simulink model "WaterTankSysIden2024"  (R2023b)
settings: Solver=FixedStepAuto  StartTime=0.0  StopTime=2000  FixedStep=0.75  RelTol=1e-3  EnableMultiTasking=on
StopFcn:
  | FileName=' SysIdenData00.mat';
  | [fPath, fName, fExt] = fileparts(FileName);
  | if isempty(fExt)  % No '.mat' in FileName
  |     fExt     = '.mat';
  |     FileName = fullfile(fPath, [fName, fExt]);
  | end
  | if exist(FileName, 'file')
  |     % Get number of files:
  |     fDir     = dir(fullfile(fPath, [fName, '*', fExt]));
  |     fStr     = lower(sprintf('%s*', fDir.name));
  |     %fNum     = sscanf(fStr, [fName, '%d', fExt, '*']);
  |     digit =  str2double(extract(fStr, digitsPattern));
  |     %newNum = digit + 1;
  |     if isempty(digit)
  |         newNum = 1;
  |     else
  |         newNum = digit + 1;
  |     end
  |     FileName = fullfile(fPath, [fName, sprintf('%d', newNum(end)), fExt]);
  | end
  | save(FileName, 'LogData');
  | clear digit fDir fExt FileName fName fPath fStr newNum fNum
undefined symbols (not defined in the file or in its folder): National_Instruments, PCIe
libraries: sldrtlib x4, simulink x1
settings Model: SimulationMode=external  ExtModeTrigDuration=7200  ExtModeArchiveMode=auto  ExtModeArchiveFileName=SysIdenData  ExtModeArchiveDirName=C:\Users\My Project\Documents\MATLAB  ExtModeAutoIncOneShot=on  ExtModeWriteAllDataToWs=on  Creator=My Project  LastModifiedBy=My Project
settings SolverCC: AlgebraicLoopSolver=TrustRegion
settings DataIOCC: LimitDataPoints=on  ReturnWorkspaceOutputs=off
settings OptimizationCC: ReuseModelBlockBuffer=off  LifeSpan=inf
settings DebuggingCC: UnconnectedInputMsg=warning  UnconnectedOutputMsg=warning  UnconnectedLineMsg=warning  AllowSymbolicDim=off  SFUnexpectedBacktrackingDiag=warning  SFNoUnconditionalDefaultTransitionDiag=warning  SFExecutionAtInitializationDiag=none  ArithmeticOperatorsInVariantConditions=warning
settings HardwareCC: ProdBitPerLong=64  ProdHWDeviceType=Intel->x86-64 (Linux 64)  TargetBitPerLong=64  TargetBitPerPointer=64  TargetIntDivRoundTo=Zero  TargetEndianess=LittleEndian  TargetWordSize=64  TargetHWDeviceType=Intel->x86-64
settings ModelReferenceCC: EnableRefExpFcnMdlSchedulingChecks=on  PropagateSignalLabelsOutOfModel=off
settings SFSimCC: SimUseLocalCustomCode=off  CustomCodeUndefinedFunction=UseInterfaceOnly
settings RTWCC: Description=Simulink Desktop Real-Time  SystemTargetFile=sldrt.tlc  TemplateMakefile=sldrt.tmf  RTWUseLocalCustomCode=off  RTWCompilerOptimization=on
settings CodeAppCC: MaxIdLength=95  StateflowObjectComments=on
settings SimulinkDesktopRealTimeCC: TargetLibSuffix=_sldrt.a  TargetPreCompLibLocation=C:\Program Files\MATLAB\R2023b\toolbox\sldrt\lib\win64  TargetLangStandard=C89/C90 (ANSI)  SupportVariableSizeSignals=off
settings ConfigComp: CovMetricSettings=dw  CovSaveCumulativeToWorkspaceVar=on  CovSaveSingleToWorkspaceVar=on  CovExternalEMLEnable=off

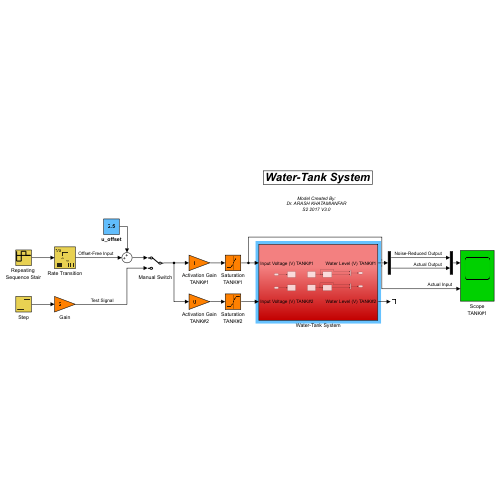
[thumbnail: Simulink's stored preview of the top-level diagram]
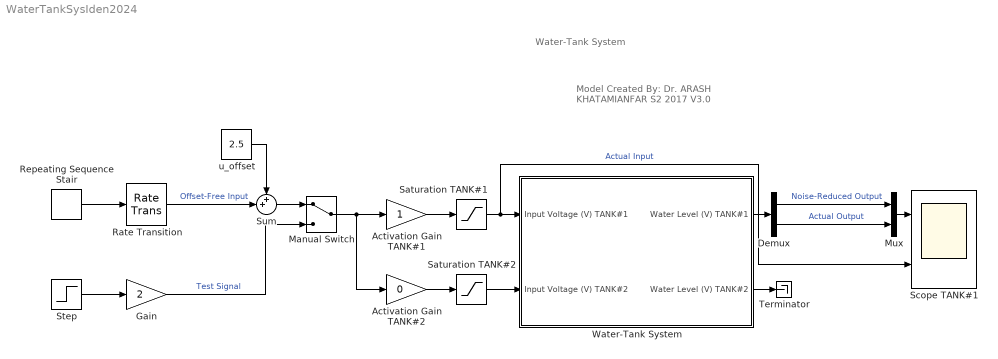
== system WaterTankSysIden2024 ==
  note: Model Created By:
      | Dr. ARASH KHATAMIANFAR
      | S2 2017 V3.0
  note: Water-Tank System
  Activation Gain TANK#1 : Gain
  Activation Gain TANK#2 : Gain  Gain=0
  Demux : Demux  Outputs=2
  Gain : Gain  Gain=2
  Manual Switch : ManualSwitch
  Mux : Mux  Inputs=2
  Rate Transition : RateTransition  OutPortSampleTime=0.75
  Repeating Sequence Stair : simulink/Sources/Repeating Sequence Stair  OutValues=[-0.3 0.2 0].'  tsamp=230*0.75  OutMin=[]  OutMax=[]  OutDataTypeStr=double  OutputDataTypeScalingMode=double  OutDataType=fixdt(0,8)  ConRadixGroup=Best Precision: Vector-wise  OutScaling=2^-12
  Saturation TANK#1 : Saturate  UpperLimit=3  LowerLimit=0
  Saturation TANK#2 : Saturate  UpperLimit=5  LowerLimit=0
  Scope TANK#1 : Scope  NumInputPorts=2
  Step : Step  Time=0  SampleTime=0
  Sum : Sum  Inputs=++|
  Terminator : Terminator
  Water-Tank System : Subsystem
  u_offset : Constant  Value=2.5
  wires:
  Step/1 -> Gain/1
  Repeating Sequence Stair/1 -> Rate Transition/1
  u_offset/1 -> Sum/1
  Sum/1 -> Manual Switch/1
  Saturation TANK#1/1 -> Water-Tank System/1(Input Voltage (V) TANK#1), Scope TANK#1/2  "Actual Input"
  Activation Gain TANK#1/1 -> Saturation TANK#1/1
  Activation Gain TANK#2/1 -> Saturation TANK#2/1
  Saturation TANK#2/1 -> Water-Tank System/2(Input Voltage (V) TANK#2)
  Rate Transition/1 -> Sum/2  "Offset-Free Input"
  Gain/1 -> Manual Switch/2  "Test Signal"
  Manual Switch/1 -> Activation Gain TANK#2/1, Activation Gain TANK#1/1
  Water-Tank System/2(Water Level (V) TANK#2) -> Terminator/1
  Water-Tank System/1(Water Level (V) TANK#1) -> Demux/1
  Demux/2 -> Mux/2  "Actual Output"
  Demux/1 -> Mux/1  "Noise-Reduced Output"
  Mux/1 -> Scope TANK#1/1

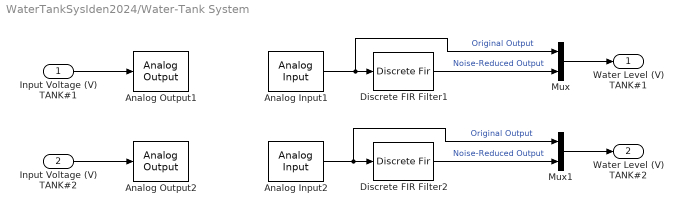
== system WaterTankSysIden2024/Water-Tank System ==
  Input Voltage (V) TANK#1 : Inport
  Input Voltage (V) TANK#2 : Inport  Port=2
  Analog Input1 : sldrtlib/Analog Input  SampleTime=0.75  MaxMissedTicks=10  ShowMissedTicks=off  YieldWhenWaiting=off  DrvName=National_Instruments/PCIe-6351  DrvAddress=4294967295  DrvOptions=[0 0 0 0 0 0 0]  Channels=1  RangeMode=1  VoltRange=1  DataType=1
      settings: AttributesFormatString=National Instruments\nPCIe-6351 [auto]
  Analog Input2 : sldrtlib/Analog Input  SampleTime=0.75  MaxMissedTicks=10  ShowMissedTicks=off  YieldWhenWaiting=off  DrvName=National_Instruments/PCIe-6351  DrvAddress=4294967295  DrvOptions=[0 0 0 0 0 0 0]  Channels=2  RangeMode=1  VoltRange=1  DataType=1
      settings: AttributesFormatString=National Instruments\nPCIe-6351 [auto]
  Analog Output1 : sldrtlib/Analog Output  SampleTime=0.75  MaxMissedTicks=10  ShowMissedTicks=off  YieldWhenWaiting=off  DrvName=National_Instruments/PCIe-6351  DrvAddress=4294967295  DrvOptions=[0 0 0 0 0 0 0]  Channels=1  RangeMode=1  VoltRange=1  InitialValue=0  FinalValue=0
      settings: AttributesFormatString=National Instruments\nPCIe-6351 [auto]
  Analog Output2 : sldrtlib/Analog Output  SampleTime=0.75  MaxMissedTicks=10  ShowMissedTicks=off  YieldWhenWaiting=off  DrvName=National_Instruments/PCIe-6351  DrvAddress=4294967295  DrvOptions=[0 0 0 0 0 0 0]  Channels=2  RangeMode=1  VoltRange=1  InitialValue=0  FinalValue=0
      settings: AttributesFormatString=National Instruments\nPCIe-6351 [auto]
  Discrete FIR Filter1 : DiscreteFir  Coefficients=[0.2 0.2 0.2 0.2 0.2]  SampleTime=0.75
  Discrete FIR Filter2 : DiscreteFir  Coefficients=[0.2 0.2 0.2 0.2 0.2]  SampleTime=0.75
  Mux : Mux  Inputs=2
  Mux1 : Mux  Inputs=2
  Water Level (V) TANK#1 : Outport
  Water Level (V) TANK#2 : Outport  Port=2
  wires:
  Analog Input1/1 -> Mux/1, Discrete FIR Filter1/1  "Original Output"
  Input Voltage (V) TANK#1/1 -> Analog Output1/1
  Discrete FIR Filter1/1 -> Mux/2  "Noise-Reduced Output"
  Mux/1 -> Water Level (V) TANK#1/1
  Analog Input2/1 -> Mux1/1, Discrete FIR Filter2/1  "Original Output"
  Input Voltage (V) TANK#2/1 -> Analog Output2/1
  Discrete FIR Filter2/1 -> Mux1/2  "Noise-Reduced Output"
  Mux1/1 -> Water Level (V) TANK#2/1
